simulink model "test_regler_polbvg_aktoren_sensoren_ansprechen"  (R2016b)
settings: Solver=ode1  StartTime=0.0  StopTime=Inf  FixedStep=0.001  RelTol=1e-3
PostLoadFcn:
  | , if any(exist('dsrtsu_mdlpostloadfcn', 'file') == [2, 3, 6]), try dsrtsu_mdlpostloadfcn('Execute', bdroot); catch fprintf('Error in PostLoadFcn (dsrtsu_mdlpostloadfcn) for model "%s":\n %s\n', bdroot, lasterr); end, end,
undefined symbols (not defined in the file): A_b_angle, A_D, B_b_angle, B_D, C_b_angle, C_D, Continuous, D_b_angle, D_D, matA_g, matA_hub_g, matB, matB_g, matB_hub, matB_hub_g, matC_g, matC_hub_g, matE, matE_hub, matR_ges, matR_hub, reglerhub, system, Time
libraries: rti1202lib_adc_class1 x3, rti1202lib_dac_class1 x2, ctrlSharedLib x2, simulink x1, rtiemclib x1, rti1202lib_base x1
(part 1 of 2)
PreSaveFcn:
  | , if any(exist('dsmpb_private', 'file') == [2, 3, 6]), try, dsmpb_private('dsmpb_mdlclblib', 'PreSave', bdroot); catch, disp(lasterr); end, end,
CloseFcn:
  | , if any(exist('dsmpb_private', 'file') == [2, 3, 6]), try, dsmpb_private('dsmpb_mdlclblib', 'Close', bdroot); catch, disp(lasterr); end, end,
settings Model: DSRTSU_INTERNAL_RTI_VER=490  DSRTSU_INTERNAL_RTI_TYPE=rti1202  DSRTSU_INTERNAL_RTIFPGA=80  DSMPB_DATASERVER_ModelPortLibVersion1=8  DSMPB_DATASERVER_DataServerVersion1=6  DSMPB_DATASERVER_DataServerStreamVersion1=3  ParamWorkspaceSource=ReferencedWorkspace  Creator=verladebruecke  LastModifiedBy=nicol
settings OptimizationCC: BlockReduction=off  OptimizeBlockIOStorage=off  BufferReuse=off  GlobalBufferReuse=off  ExpressionFolding=off  LocalBlockOutputs=off
settings HardwareCC: ProdBitPerPointer=32  ProdBitPerSizeT=32  ProdBitPerPtrDiffT=32  ProdLargestAtomicInteger=Integer  ProdEndianess=BigEndian  ProdWordSize=32  ProdHWDeviceType=Custom Processor->Custom  TargetIntDivRoundTo=Zero  TargetEndianess=BigEndian  TargetHWDeviceType=Custom Processor->Custom
settings RTWCC: SystemTargetFile=rti1202.tlc  MakeCommand=make_rti  TemplateMakefile=rti1202.tmf  Description=dSPACE DS1202 Hardware Platform
settings STFCustomTargetCC: ParMdlRefBuildCompliant=on  GRTInterface=off  SystemTargetFile=rti1202.tlc
settings GRTTargetCC: TargetLangStandard=C89/C90 (ANSI)  CompOptLevelCompliant=off  ConcurrentExecutionCompliant=off  CombineOutputUpdateFcns=off  MatFileLogging=off  CPPClassGenCompliant=off  UseToolchainInfoCompliant=off
settings ConfigComp: CovMetricSettings=dswe

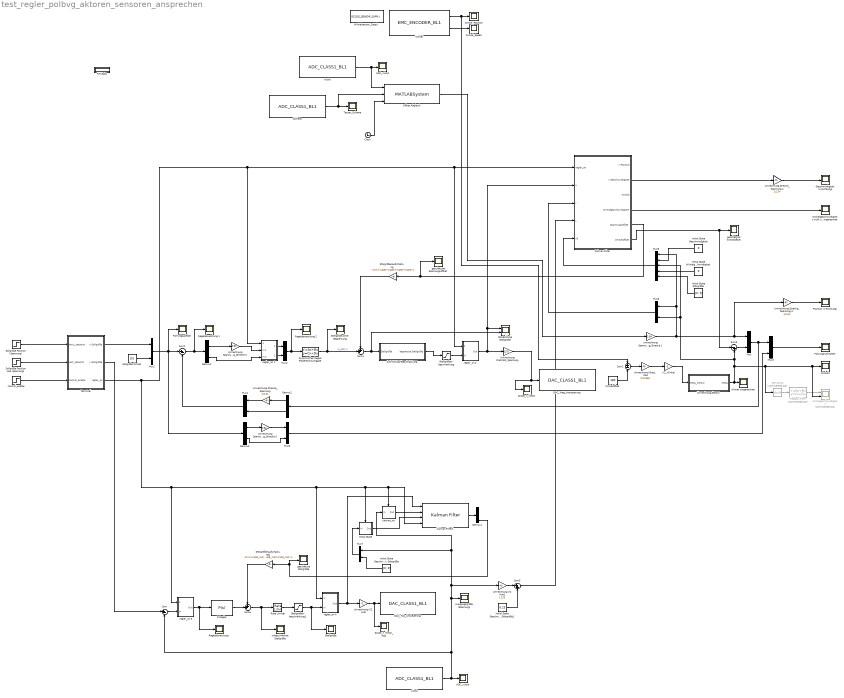
== system test_regler_polbvg_aktoren_sensoren_ansprechen ==
  ADC_xUout : Scope
  ADC_yUout : Scope
  Anti-Schlupf Beschränkung : Subsystem
  Ausgangsgröße (Spannung) : Scope
  Clock : Clock
  DAC_Hub_Ansteuerung : rti1202lib_dac_class1/DAC_CLASS1_BL1  DSProperties=struct('RTI',struct('Version',uint32(2),'BlockType',struct('isSLSource',uint8(0),'isSLSink',uint8(1),'isHWSource',uint8(0),'isHWSink',uint8(1),'isSetup',uint8(0),'isInline',uint8(1),'isNonInline',uint8(0),'isInterrupt',uint8(0),'isChannelwise',uint8(1)),'IOBoardType',{{'DS120X','STD','DACC1'}},'UnitType','DAC','Identifier','DAC','DialogType','ML','BlockSet','NONE','SlaveProcessor','NONE'))  RTIBlockInterface=struct('InputPortsActive',1,'InputPortsWidth',int32(1),'InputPortsDataType',{{'SS_DOUBLE'}},'InputPortsName',{{['DAC 2']}},'DialogFcn','rti120xstddacc1dacgui','InitLevel',3,'IconTransparency','on','BlockDisplay',{{['DAC CL1\nChannel: 2'],'center'}},'BlockName',struct('Token',{{'DAC_CLASS1_BL1'}}))  RTIBlockParameters=struct('ChannelNo',{{2,'OFF',[]}},'ChannelNumOf',{{1,'OFF',[]}},'InitialValue1',{{'0','OFF',[-10 10]}},'InitialValue2',{{'0','OFF',[-10 10]}},'InitialValue3',{{'0','OFF',[-10 10]}},'InitialValue4',{{'0','OFF',[-10 10]}},'InitialValue5',{{'0','OFF',[-10 10]}},'InitialValue6',{{'0','OFF',[-10 10]}},'InitialValue7',{{'0','OFF',[-10 10]}},'InitialValue8',{{'0','OFF',[-10 10]}},'InitialValue9',{{'0','OFF',[-10 10]}},'InitialValue10',{{'0','OFF',[-10 10]}},'InitialValue11',{{'0','OFF',[-10 10]}},'InitialValue12',{{'0','OFF',[-10 10]}},'InitialValue13',{{'0','OFF',[-10 10]}},'InitialValue14',{{'0','OFF',[-10 10]}},'InitialValue15',{{'0','OFF',[-10 10]}},'InitialValue16',{{'0','OFF',[-10 10]}},'OutputMode',{{[1 1 1 1 1 1 1 1 1 1 1 1 1 1 1 1],'OFF',[1 2]}},'TermValue1',{{'0','OFF',[-10 10]}},'TermValue2',{{'0','OFF',[-10 10]}},'TermValue3',{{'0','OFF',[-10 10]}},'TermValue4',{{'0','OFF',[-10 10]}},'TermValue5',{{'0','OFF',[-10 10]}},'TermValue6',{{'0','OFF',[-10 10]}},'TermValue7',{{'0','OFF',[-10 10]}},'TermValue8',{{'0','OFF',[-10 10]}},'TermValue9',{{'0','OFF',[-10 10]}},'TermValue10',{{'0','OFF',[-10 10]}},'TermValue11',{{'0','OFF',[-10 10]}},'TermValue12',{{'0','OFF',[-10 10]}},'TermValue13',{{'0','OFF',[-10 10]}},'TermValue14',{{'0','OFF',[-10 10]}},'TermValue15',{{'0','OFF',[-10 10]}},'TermValue16',{{'0','OFF',[-10 10]}},'EnableTermMode',{{0,'OFF',[0 1]}},'TLCFileName',{{'rti120xdac_c1_dac','OFF',[]}},'InitialValueBuildCheck1',{{0,'OFF',[]}},'InitialValueBuildCheck2',{{1,'OFF',[]}},'InitialValueBuildCheck3',{{0,'OFF',[]}},'InitialValueBuildCheck4',{{0,'OFF',[]}},'InitialValueBuildCheck5',{{0,'OFF',[]}},'InitialValueBuildCheck6',{{0,'OFF',[]}},'InitialValueBuildCheck7',{{0,'OFF',[]}},'InitialValueBuildCheck8',{{0,'OFF',[]}},'InitialValueBuildCheck9',{{0,'OFF',[]}},'InitialValueBuildCheck10',{{0,'OFF',[]}},'InitialValueBuildCheck11',{{0,'OFF',[]}},'InitialValueBuildCheck12',{{0,'OFF',[]}},'InitialValueBuildCheck13',{{0,'OFF',[]}},'InitialValueBuildCheck14',{{0,'OFF',[]}},'InitialValueBuildCheck15',{{0,'OFF',[]}},'InitialValueBuildCheck16',{{0,'OFF',[]}},'TermValueBuildCheck1',{{0,'OFF',[]}},'TermValueBuildCheck2',{{0,'OFF',[]}},'TermValueBuildCheck3',{{0,'OFF',[]}},'TermValueBuildCheck4',{{0,'OFF',[]}},'TermValueBuildCheck5',{{0,'OFF',[]}},'TermValueBuildCheck6',{{0,'OFF',[]}},'TermValueBuildCheck7',{{0,'OFF',[]}},'TermValueBuildCheck8',{{0,'OFF',[]}},'TermValueBuildCheck9',{{0,'OFF',[]}},'TermValueBuildCheck10',{{0,'OFF',[]}},'TermValueBuildCheck11',{{0,'OFF',[]}},'TermValueBuildCheck12',{{0,'OFF',[]}},'TermValueBuildCheck13',{{0,'OFF',[]}},'TermValueBuildCheck14',{{0,'OFF',[]}},'TermValueBuildCheck15',{{0,'OFF',[]}},'TermValueBuildCheck16',{{0,'OFF',[]}})  RTISFcnParameters=struct('ChannelNo','int16','ChannelNumOf','int16','InitialValue1','double','InitialValue2','double','InitialValue3','double','InitialValue4','double','InitialValue5','double','InitialValue6','double','InitialValue7','double','InitialValue8','double','InitialValue9','double','InitialValue10','double','InitialValue11','double','InitialValue12','double','InitialValue13','double','InitialValue14','double','InitialValue15','double','InitialValue16','double','OutputMode','int16','TermValue1','double','TermValue2','double','TermValue3','double','TermValue4','double','TermValue5','double','TermValue6','double','TermValue7','double','TermValue8','double','TermValue9','double','TermValue10','double','TermValue11','double','TermValue12','double','TermValue13','double','TermValue14','double','TermValue15','double','TermValue16','double','EnableTermMode','int16','TLCFileName','char')  RTIBlockParaDefault=struct('ChannelNo',1,'ChannelNumOf',1,'InitialValue1',0,'InitialValue2',0,'InitialValue3',0,'InitialValue4',0,'InitialValue5',0,'InitialValue6',0,'InitialValue7',0,'InitialValue8',0,'InitialValue9',0,'InitialValue10',0,'InitialValue11',0,'InitialValue12',0,'InitialValue13',0,'InitialValue14',0,'InitialValue15',0,'InitialValue16',0,'OutputMode',[1 1 1 1 1 1 1 1 1 1 1 1 1 1 1 1],'TermValue1',0,'TermValue2',0,'TermValue3',0,'TermValue4',0,'TermValue5',0,'TermValue6',0,'TermValue7',0,'TermValue8',0,'TermValue9',0,'TermValue10',0,'TermValue11',0,'TermValue12',0,'TermValue13',0,'TermValue14',0,'TermValue15',0,'TermValue16',0,'EnableTermMode',0,'TLCFileName','rti120xdac_c1_dac','InitialValueBuildCheck1',0,'InitialValueBuildCheck2',0,'InitialValueBuildCheck3',0,'InitialValueBuildCheck4',0,'InitialValueBuildCheck5',0,'InitialValueBuildCheck6',0,'InitialValueBuildCheck7',0,'InitialValueBuildCheck8',0,'InitialValueBuildCheck9',0,'InitialValueBuildCheck10',0,'InitialValueBuildCheck11',0,'InitialValueBuildCheck12',0,'InitialValueBuildCheck13',0,'InitialValueBuildCheck14',0,'InitialValueBuildCheck15',0,'InitialValueBuildCheck16',0,'TermValueBuildCheck1',0,'TermValueBuildCheck2',0,'TermValueBuildCheck3',0,'TermValueBuildCheck4',0,'TermValueBuildCheck5',0,'TermValueBuildCheck6',0,'TermValueBuildCheck7',0,'TermValueBuildCheck8',0,'TermValueBuildCheck9',0,'TermValueBuildCheck10',0,'TermValueBuildCheck11',0,'TermValueBuildCheck12',0,'TermValueBuildCheck13',0,'TermValueBuildCheck14',0,'TermValueBuildCheck15',0,'TermValueBuildCheck16',0)
  DAC_Weg_Ansteuerung : rti1202lib_dac_class1/DAC_CLASS1_BL1  DSProperties=struct('RTI',struct('Version',uint32(2),'BlockType',struct('isSLSource',uint8(0),'isSLSink',uint8(1),'isHWSource',uint8(0),'isHWSink',uint8(1),'isSetup',uint8(0),'isInline',uint8(1),'isNonInline',uint8(0),'isInterrupt',uint8(0),'isChannelwise',uint8(1)),'IOBoardType',{{'DS120X','STD','DACC1'}},'UnitType','DAC','Identifier','DAC','DialogType','ML','BlockSet','NONE','SlaveProcessor','NONE'))  RTIBlockInterface=struct('InputPortsActive',1,'InputPortsWidth',int32(1),'InputPortsDataType',{{'SS_DOUBLE'}},'InputPortsName',{{['DAC 1']}},'DialogFcn','rti120xstddacc1dacgui','InitLevel',3,'IconTransparency','on','BlockDisplay',{{['DAC CL1\nChannel: 1'],'center'}},'BlockName',struct('Token',{{'DAC_CLASS1_BL1'}}))  RTIBlockParameters=struct('ChannelNo',{{1,'OFF',[]}},'ChannelNumOf',{{1,'OFF',[]}},'InitialValue1',{{0,'OFF',[-10 10]}},'InitialValue2',{{0,'OFF',[-10 10]}},'InitialValue3',{{0,'OFF',[-10 10]}},'InitialValue4',{{0,'OFF',[-10 10]}},'InitialValue5',{{0,'OFF',[-10 10]}},'InitialValue6',{{0,'OFF',[-10 10]}},'InitialValue7',{{0,'OFF',[-10 10]}},'InitialValue8',{{0,'OFF',[-10 10]}},'InitialValue9',{{0,'OFF',[-10 10]}},'InitialValue10',{{0,'OFF',[-10 10]}},'InitialValue11',{{0,'OFF',[-10 10]}},'InitialValue12',{{0,'OFF',[-10 10]}},'InitialValue13',{{0,'OFF',[-10 10]}},'InitialValue14',{{0,'OFF',[-10 10]}},'InitialValue15',{{0,'OFF',[-10 10]}},'InitialValue16',{{0,'OFF',[-10 10]}},'OutputMode',{{[1 1 1 1 1 1 1 1 1 1 1 1 1 1 1 1],'OFF',[1 2]}},'TermValue1',{{0,'OFF',[-10 10]}},'TermValue2',{{0,'OFF',[-10 10]}},'TermValue3',{{0,'OFF',[-10 10]}},'TermValue4',{{0,'OFF',[-10 10]}},'TermValue5',{{0,'OFF',[-10 10]}},'TermValue6',{{0,'OFF',[-10 10]}},'TermValue7',{{0,'OFF',[-10 10]}},'TermValue8',{{0,'OFF',[-10 10]}},'TermValue9',{{0,'OFF',[-10 10]}},'TermValue10',{{0,'OFF',[-10 10]}},'TermValue11',{{0,'OFF',[-10 10]}},'TermValue12',{{0,'OFF',[-10 10]}},'TermValue13',{{0,'OFF',[-10 10]}},'TermValue14',{{0,'OFF',[-10 10]}},'TermValue15',{{0,'OFF',[-10 10]}},'TermValue16',{{0,'OFF',[-10 10]}},'EnableTermMode',{{0,'OFF',[0 1]}},'TLCFileName',{{'rti120xdac_c1_dac','OFF',[]}},'InitialValueBuildCheck1',{{0,'OFF',[]}},'InitialValueBuildCheck2',{{0,'OFF',[]}},'InitialValueBuildCheck3',{{0,'OFF',[]}},'InitialValueBuildCheck4',{{0,'OFF',[]}},'InitialValueBuildCheck5',{{0,'OFF',[]}},'InitialValueBuildCheck6',{{0,'OFF',[]}},'InitialValueBuildCheck7',{{0,'OFF',[]}},'InitialValueBuildCheck8',{{0,'OFF',[]}},'InitialValueBuildCheck9',{{0,'OFF',[]}},'InitialValueBuildCheck10',{{0,'OFF',[]}},'InitialValueBuildCheck11',{{0,'OFF',[]}},'InitialValueBuildCheck12',{{0,'OFF',[]}},'InitialValueBuildCheck13',{{0,'OFF',[]}},'InitialValueBuildCheck14',{{0,'OFF',[]}},'InitialValueBuildCheck15',{{0,'OFF',[]}},'InitialValueBuildCheck16',{{0,'OFF',[]}},'TermValueBuildCheck1',{{0,'OFF',[]}},'TermValueBuildCheck2',{{0,'OFF',[]}},'TermValueBuildCheck3',{{0,'OFF',[]}},'TermValueBuildCheck4',{{0,'OFF',[]}},'TermValueBuildCheck5',{{0,'OFF',[]}},'TermValueBuildCheck6',{{0,'OFF',[]}},'TermValueBuildCheck7',{{0,'OFF',[]}},'TermValueBuildCheck8',{{0,'OFF',[]}},'TermValueBuildCheck9',{{0,'OFF',[]}},'TermValueBuildCheck10',{{0,'OFF',[]}},'TermValueBuildCheck11',{{0,'OFF',[]}},'TermValueBuildCheck12',{{0,'OFF',[]}},'TermValueBuildCheck13',{{0,'OFF',[]}},'TermValueBuildCheck14',{{0,'OFF',[]}},'TermValueBuildCheck15',{{0,'OFF',[]}},'TermValueBuildCheck16',{{0,'OFF',[]}})  RTISFcnParameters=struct('ChannelNo','int16','ChannelNumOf','int16','InitialValue1','double','InitialValue2','double','InitialValue3','double','InitialValue4','double','InitialValue5','double','InitialValue6','double','InitialValue7','double','InitialValue8','double','InitialValue9','double','InitialValue10','double','InitialValue11','double','InitialValue12','double','InitialValue13','double','InitialValue14','double','InitialValue15','double','InitialValue16','double','OutputMode','int16','TermValue1','double','TermValue2','double','TermValue3','double','TermValue4','double','TermValue5','double','TermValue6','double','TermValue7','double','TermValue8','double','TermValue9','double','TermValue10','double','TermValue11','double','TermValue12','double','TermValue13','double','TermValue14','double','TermValue15','double','TermValue16','double','EnableTermMode','int16','TLCFileName','char')  RTIBlockParaDefault=struct('ChannelNo',1,'ChannelNumOf',1,'InitialValue1',0,'InitialValue2',0,'InitialValue3',0,'InitialValue4',0,'InitialValue5',0,'InitialValue6',0,'InitialValue7',0,'InitialValue8',0,'InitialValue9',0,'InitialValue10',0,'InitialValue11',0,'InitialValue12',0,'InitialValue13',0,'InitialValue14',0,'InitialValue15',0,'InitialValue16',0,'OutputMode',[1 1 1 1 1 1 1 1 1 1 1 1 1 1 1 1],'TermValue1',0,'TermValue2',0,'TermValue3',0,'TermValue4',0,'TermValue5',0,'TermValue6',0,'TermValue7',0,'TermValue8',0,'TermValue9',0,'TermValue10',0,'TermValue11',0,'TermValue12',0,'TermValue13',0,'TermValue14',0,'TermValue15',0,'TermValue16',0,'EnableTermMode',0,'TLCFileName','rti120xdac_c1_dac','InitialValueBuildCheck1',0,'InitialValueBuildCheck2',0,'InitialValueBuildCheck3',0,'InitialValueBuildCheck4',0,'InitialValueBuildCheck5',0,'InitialValueBuildCheck6',0,'InitialValueBuildCheck7',0,'InitialValueBuildCheck8',0,'InitialValueBuildCheck9',0,'InitialValueBuildCheck10',0,'InitialValueBuildCheck11',0,'InitialValueBuildCheck12',0,'InitialValueBuildCheck13',0,'InitialValueBuildCheck14',0,'InitialValueBuildCheck15',0,'InitialValueBuildCheck16',0,'TermValueBuildCheck1',0,'TermValueBuildCheck2',0,'TermValueBuildCheck3',0,'TermValueBuildCheck4',0,'TermValueBuildCheck5',0,'TermValueBuildCheck6',0,'TermValueBuildCheck7',0,'TermValueBuildCheck8',0,'TermValueBuildCheck9',0,'TermValueBuildCheck10',0,'TermValueBuildCheck11',0,'TermValueBuildCheck12',0,'TermValueBuildCheck13',0,'TermValueBuildCheck14',0,'TermValueBuildCheck15',0,'TermValueBuildCheck16',0)
  Demux1 : Demux  Outputs=2
  Demux2 : Demux  Outputs=2
  Demux3 : Demux  Outputs=2
  Demux4 : Demux  Outputs=3
  Derivative : Derivative  Commented=on
  Dynamischer Regler Polbereichsvorgabe : StateSpace  A=A_D  B=-B_D  C=-C_D  D=D_D  X0=0
  Führungsgrößen : Scope
  Führungsverhalten : Scope
  Geschwindigkeit (x-Richtung) : Scope
  Initial State : Subsystem  TreatAsAtomicUnit=on
  Initial State Geschwindigkeit : Constant  Value=0  VectorParams1D=off
  "Initial State Geschwindigkeit, Störgröße" : Constant  Value=[0; 0]  VectorParams1D=off
  "Initial State Geschwindigkeit, Störgröße1" : Constant  Value=0.23  VectorParams1D=off
  Initial State Störgröße : Constant  Value=[0; 0]  VectorParams1D=off
  Initial State Winkelgeschwindigkeit : Constant  Value=0  VectorParams1D=off
  Kalman Filter : Subsystem
  Kalman Filter1 : ctrlSharedLib/Kalman Filter  TimeDomain=Continuous-Time  UseCurrentEstimator=on  ModelSource=Individual A, B, C, D matrices  ModelSourceVariable=ss(0.95,1,1,0,1)  A=matA_hub_g  B=matB_hub_g  C=matC_hub_g  D=0  NumberOfStates=1  NumberOfInputs=1  NumberOfOutputs=1  InitialEstimateSource=Input port  X0=0  P0=10  UseK=off  UseGH=on  NumberOfProcessNoiseInputs=1  G=matG_hub  TimeInvariantG=on  H=0  TimeInvariantH=on  Q=matQ_hub  TimeInvariantQ=on  R=matR_hub  TimeInvariantR=on  N=0  TimeInvariantN=on  AddInputPort=on  AddEnablePort=off  ExternalReset=rising  OutputEstimatedY=off  OutputP=off  Ts=-1
  Mux{,1..5,7..8} (8 alike) : Mux  Inputs=2
  Mux6 : Mux  Inputs=5
  Offset Abgleich : MATLABSystem  System=offset_abgleich  SimulateUsing=Code generation
      mask Type: offset_abgleich
      mask Display:
      | disp('offset_abgleich');
      | port_label('input',1,'input');
      | port_label('input',2,'taster');
      | port_label('input',3,'clock');
      | port_label('output',1,'output');
  P-Regler : simulink/Continuous/PID Controller  Controller=P  TimeDomain=Continuous-time  SampleTime=-1  IntegratorMethod=Forward Euler  FilterMethod=Forward Euler  Form=Parallel  UseFilter=on  ControllerParametersSource=internal  P=reglerhub.P  I=0  D=0.1  N=100  InitialConditionSource=internal  InitialConditionForIntegrator=0  InitialConditionForFilter=0  ExternalReset=falling  LimitOutput=off  UpperSaturationLimit=inf  LowerSaturationLimit=-inf  LinearizeAsGain=on  AntiWindupMode=none  Kb=1  TrackingMode=on  Kt=2  PParamMin=[]  PParamMax=[]  IParamMin=[]  IParamMax=[]  DParamMin=[]  DParamMax=[]  NParamMin=[]  NParamMax=[]  KbParamMin=[]  KbParamMax=[]  KtParamMin=[]  KtParamMax=[]  POutMin=[]  POutMax=[]  IOutMin=[]  IOutMax=[]  DOutMin=[]  DOutMax=[]  NOutMin=[]  NOutMax=[]  KbOutMin=[]  KbOutMax=[]  KtOutMin=[]  KtOutMax=[]  IntegratorOutMin=[]  IntegratorOutMax=[]  FilterOutMin=[]  FilterOutMax=[]  SumOutMin=[]  SumOutMax=[]  SumI1OutMin=[]  SumI1OutMax=[]  SumI2OutMin=[]  SumI2OutMax=[]  SumI3OutMin=[]  SumI3OutMax=[]  SumDOutMin=[]  SumDOutMax=[]  SaturationOutMin=[]  SaturationOutMax=[]  IntegratorContinuousStateAttributes=''  IntegratorStateMustResolveToSignalObject=off  IntegratorRTWStateStorageClass=Auto  FilterContinuousStateAttributes=''  FilterStateMustResolveToSignalObject=off  FilterRTWStateStorageClass=Auto  DifferentiatorICPrevScaledInput=0  DifferentiatorOutMin=[]  DifferentiatorOutMax=[]
  Position (x-Richtung) : Scope
  RTI Data : Subsystem  Tag=struct('RTIDataServer',struct('RTIDataServerVs','2','RTIModelDescription','struct(''main'',''aktoren_sensoren_ansprechen'',''sub'','''',''isMp'',0)'))  LoadFcn="if exist('rtidc'), try,  rtidc('DataHostBlockClbLoad', gcbh); catch, disp(['Warning: ''LoadFcn'' for RTI Data block failed: ' lasterr]); end, end,"  mask(RTI_DATA_HOST){}
      mask help:
      | RTI Data Block.
      | This block is used by RTI to store internal model-dependent data.
      | Please keep this block on the root level of the model. Deleting this block will result in data loss.
      |
      | NEVER DELETE OR COPY THIS BLOCK!
      settings: CopyFcn="if exist('rtidc'), try,  rtidc('DataHostBlockClbCopy', gcbh); catch, disp(['Warning: ''CopyFcn'' for RTI Data block failed: ' lasterr]); end, end,"  DeleteFcn="if exist('rtidc'), try,  rtidc('DataHostBlockClbDelete', gcbh); catch, disp(['Warning: ''DeleteFcn'' for RTI Data block failed: ' lasterr]); end, end,"  ModelCloseFcn="if exist('rtidc'), try,  rtidc('DataHostBlockClbModelClose', gcbh); catch, disp(['Warning: ''ModelCloseFcn'' for RTI Data block failed: ' lasterr]); end, end,"  PreSaveFcn="if exist('rtidc'), try,  rtidc('DataHostBlockClbPreSave', gcbh); catch, disp(['Warning: ''PreSaveFcn'' for RTI Data block failed: ' lasterr]); end, end,"  PostSaveFcn="if exist('rtidc'), try,  rtidc('DataHostBlockClbPostSave', gcbh); catch, disp(['Warning: ''PostSaveFcn'' for RTI Data block failed: ' lasterr]); end, end,"  NameChangeFcn="if exist('rtidc'), try,  rtidc('DataHostBlockClbNameChange', gcbh); catch, disp(['Warning: ''NameChangeFcn'' for RTI Data block failed: ' lasterr]); end, end,"
      mask Help:
      | RTI Data Block.
      | This block is used by RTI to store internal model-dependent data.
      | Please keep this block on the root level of the model. Deleting this block will result in data loss.
      | 
      | NEVER DELETE OR COPY THIS BLOCK!
      mask Display:
      | text(0.5, 0.5, 'RTI Data', 'HorizontalAlignment', 'center');
      | plot([1 0]);
  Rate Limiter : RateLimiter  RisingSlewLimit=0.23024  FallingSlewLimit=-0.23024  SampleTimeMode=inherited
  Regelabweichung : Scope
  Regelabweichung 1 : Scope
  Regelabweichung 2 : Scope
  Schiene : rti1202lib_adc_class1/ADC_CLASS1_BL1  DSProperties=struct('RTI',struct('Version',uint32(1),'BlockType',struct('isSLSource',uint8(1),'isSLSink',uint8(1),'isHWSource',uint8(0),'isHWSink',uint8(1),'isSetup',uint8(0),'isInline',uint8(1),'isNonInline',uint8(0),'isInterrupt',uint8(0),'isChannelwise',uint8(1)),'IOBoardType',{{'DS120X','STD','ADCC1'}},'UnitType','ADC','Identifier','ADC','DialogType','ML','BlockSet','NONE','SlaveProcessor','NONE'))  RTIBlockInterface=struct('InputPortsActive',0,'InputPortsWidth',int32(1),'InputPortsDataType',{{'SS_BOOLEAN'}},'InputPortsName',{{'Continue'}},'OutputPortsActive',[1 0],'OutputPortsWidth',int32([1 1]),'OutputPortsDataType',{{'SS_DOUBLE','SS_INT16'}},'OutputPortsName',{{'ADC','Status'}},'DialogFcn','rti120xstdadcc1adcgui','SampleTime',{{-1}},'InitLevel',3,'IconTransparency','on','BlockDisplay',{{['ADC CL1\nChannel: 10'],'center'}},'BlockName',struct('Token',{{'ADC_CLASS1_BL1'}}))  RTIBlockParameters=struct('ReadMode',{{1,'OFF',[1 2]}},'ChannelNo',{{10,'OFF',[]}},'ConversionMode',{{1,'OFF',[1 2]}},'TriggerSource',{{1,'OFF',[1 2]}},'TriggerLineIn',{{1,'OFF',[1 16]}},'SampleMode',{{1,'OFF',[1 2]}},'BurstTriggerSource',{{1,'OFF',[1 2]}},'BurstTriggerLine',{{1,'OFF',[1 16]}},'ConvTriggerSource',{{3,'OFF',[1 3]}},'ConvTriggerLine',{{1,'OFF',[1 16]}},'ConvPeriod',{{'100e-6','OFF',[1e-06 1.34]}},'ConvPeriodCheck',{{0,'OFF',[]}},'BurstSize',{{'10','OFF',[]}},'BurstSizeCheck',{{0,'OFF',[]}},'DataSetOffset',{{'0','OFF',[]}},'DataSetOffsetCheck',{{0,'OFF',[]}},'DataSetLength',{{'1','OFF',[]}},'DataSetLengthCheck',{{0,'OFF',[]}},'EnableTriggerEvent',{{0,'OFF',[0 1]}},'TriggerMode',{{2,'OFF',[1 3]}},'TriggerLineOut',{{1,'OFF',[1 16]}},'ADCSWStartEnable',{{0,'OFF',[0 1]}},'SampleTime',{{'-1','OFF',[-1 inf]}},'SampleTimeCheck',{{1,'OFF',[]}},'StatusPortEnable',{{0,'OFF',[0 1]}},'TLCFileName',{{'rti120xadc_c1_adc','OFF',[]}})  RTISFcnParameters=struct('ReadMode','int16','ChannelNo','int16','ConversionMode','int16','TriggerSource','int16','TriggerLineIn','int16','SampleMode','int16','BurstTriggerSource','int16','BurstTriggerLine','int16','ConvTriggerSource','int16','ConvTriggerLine','int16','ConvPeriod','double','BurstSize','int16','DataSetOffset','int16','DataSetLength','int16','EnableTriggerEvent','int16','TriggerMode','int16','TriggerLineOut','int16','ADCSWStartEnable','int16','SampleTime','double','StatusPortEnable','int16','TLCFileName','char')  RTIBlockParaDefault=struct('ReadMode',1,'ChannelNo',1,'ConversionMode',1,'TriggerSource',1,'TriggerLineIn',1,'SampleMode',1,'BurstTriggerSource',1,'BurstTriggerLine',1,'ConvTriggerSource',3,'ConvTriggerLine',1,'ConvPeriod',0.0001,'ConvPeriodCheck',0,'BurstSize',10,'BurstSizeCheck',0,'DataSetOffset',0,'DataSetOffsetCheck',0,'DataSetLength',1,'DataSetLengthCheck',0,'EnableTriggerEvent',0,'TriggerMode',2,'TriggerLineOut',1,'ADCSWStartEnable',0,'SampleTime',-1,'SampleTimeCheck',1,'StatusPortEnable',0,'TLCFileName','rti120xadc_c1_adc')
  Scope_n_Motor : Scope
  Scope_n_Motor_Hub : Scope
  Sollgröße Position (Spannung) : Step  Time=2  SampleTime=0
  Sollgröße Position Hub (Spannung) : Step  Time=2  After=0.5  SampleTime=0
  Sollgröße Winkel : Constant  Value=[0]  VectorParams1D=off
  Stellgröße : Scope
  Stellgröße ohne Begrenzung : Scope
  Stellgrößen- beschränkung : Saturate  UpperLimit=75  LowerLimit=-75
  Stellgrößen- beschränkung1 : Saturate  UpperLimit=1  LowerLimit=-1
  Störgrößenaufschaltung : Gain  Gain=-1*inv(matB'*matB)*matB'*matE  Multiplication=Matrix(K*u)
  Störgrößenaufschaltung1 : Gain  Gain=-1*inv(matB_hub'*matB_hub)*matB_hub'*matE_hub  Multiplication=Matrix(K*u)
  Sum : Sum  Inputs=|+-
  Sum1 : Sum  Inputs=|+-
  Sum2 : Sum  Inputs=+|-
  Sum3 : Sum  Inputs=|-+
  Sum4 : Sum  Inputs=++|
  Sum5 : Sum  Inputs=|++
  Sum6 : Sum  Inputs=++|
  Taster_Schiene : Scope
  Terminal : Subsystem
  Tiefpass Filter : StateSpace  Commented=on  A=A_b_angle  B=B_b_angle  C=C_b_angle  D=D_b_angle  X0=0
  Umrechnung Drehzahl_Spannung : Gain  Gain=1/75
  Umrechnung Grad_Rad : Gain  Gain=2*pi/360
  Umrechnung Spannung_Strecke 1 : Gain  Gain=2.54
  Umrechnung Spannung_Strecke 2 : Gain  Gain=2.54
  Umrechnung Spannung_Strecke 3 : Gain  Gain=2.54
  Umrechnung Strecke_Spannung : Gain  Gain=1/2.54
  Umrechnung Strecke_Spannung 3 : Gain  Gain=1/2.54
  Umrechnung Strecke_Spannung 4 : Gain  Gain=1/2.54
  Umrechnung VZ Hub : Gain  Gain=-1
  Umrechnung VZ Hub1 : Gain  Gain=1.375
  Umrechnung Sensor : MATLAB Function  TreatAsAtomicUnit=on
  VZ_Winkel : Gain  Gain=-1
  Winkel : rtiemclib/EMC_ENCODER_BL1  DSProperties=struct('RTI',struct('Version',uint32(1),'BlockType',struct('isSLSource',uint8(1),'isSLSink',uint8(0),'isHWSource',uint8(1),'isHWSink',uint8(0),'isSetup',uint8(0),'isInline',uint8(1),'isNonInline',uint8(0),'isInterrupt',uint8(0),'isChannelwise',uint8(1)),'IOBoardType','DSEMC','UnitType','ENCODER','Identifier','ENCODER','DialogType','ML','BlockSet','RTIEMC','SlaveProcessor','NONE'))  RTIBlockInterface=struct('OutputPortsWidth',int32([1 1 1]),'OutputPortsActive',int32([1 1 0]),'OutputPortsName',{{'Position','Speed',['Index Detected']}},'OutputPortsDataType',{{'SS_DOUBLE','SS_DOUBLE','SS_BOOLEAN'}},'InitLevel',3,'IconTransparency','on','BlockDisplay',{{['EMC Encoder\nUnit: 1\nDIO class: 2\nPort: 1\nChannel: 1'],'center'}},'DialogFcn','rtiemcencodergui','BlockName',struct('Token',{{'EMC_ENCODER_BL1'}}))  RTIBlockParameters=struct('UnitNo',{{1,'OFF',[1 6]}},'DioClassNo',{{2,'OFF',[1 2]}},'PortNo',{{1,'OFF',[1 1]}},'ChannelNo',{{1,'OFF',[1 11]}},'HwSignalPin',{{['DIO1 ch1'],'OFF',[]}},'HwRefPin',{{'GND','OFF',[]}},'EnablePosMeasurement',{{0,'OFF',[0 1]}},'IndexSetMode',{{1,'OFF',[1 3]}},'NumOfLines',{{'1024','OFF',[1 2097152]}},'InitAngleValue',{{'180','OFF',[0 359.99999]}},'IndexAngleValue',{{'0','OFF',[0 359.99999]}},'MinPosValue',{{'0','OFF',[-2097152 2097150.75]}},'MaxPosValue',{{'1023.75','OFF',[-2097151 2097151.75]}},'InitPosValue',{{'0','OFF',[-2097152 2097151.75]}},'IndexPosValue',{{'0','OFF',[-2097152 2097151.75]}},'IndexGateMode',{{0,'OFF',[0 1]}},'EnableNoiseFilter',{{0,'OFF',[0 1]}},'FilterInterval',{{'0','OFF',[0 0.01]}},'IndexDetectedOutPortMode',{{0,'OFF',[0 1]}},'BuildCheckAngleMeasurement',{{1,'OFF',[0 1]}},'BuildCheckAngleIndexMode',{{0,'OFF',[0 1]}},'BuildCheckPosIndexMode',{{0,'OFF',[0 1]}},'TLCFileName',{{'rtiemcencoder','OFF',[]}})  RTISFcnParameters=struct('UnitNo','int32','DioClassNo','int32','PortNo','int32','ChannelNo','int32','EnablePosMeasurement','int32','IndexSetMode','int32','IndexDetectedOutPortMode','int32','NumOfLines','uint32','InitAngleValue','double','IndexAngleValue','double','MinPosValue','double','MaxPosValue','double','InitPosValue','double','IndexPosValue','double','IndexGateMode','int32','EnableNoiseFilter','int32','FilterInterval','double','TLCFileName','char')  RTIBlockParaDefault=struct('UnitNo',1,'DioClassNo',1,'PortNo',1,'ChannelNo',1,'HwSignalPin',['DIO1 ch1'],'HwRefPin','GND','EnablePosMeasurement',0,'IndexSetMode',1,'NumOfLines',1024,'InitAngleValue',60,'IndexAngleValue',0,'MinPosValue',0,'MaxPosValue',1023.75,'InitPosValue',0,'IndexPosValue',0,'IndexGateMode',0,'EnableNoiseFilter',0,'FilterInterval',0,'IndexDetectedOutPortMode',0,'BuildCheckAngleMeasurement',0,'BuildCheckAngleIndexMode',0,'BuildCheckPosIndexMode',0,'TLCFileName','rtiemcencoder')
  Winkel umgerechnet : Scope
  Winkel1 : Scope
  Winkel_Position : Scope
  Winkel_Speed : Scope
  Winkelgeschwindigkeit : Scope  Commented=on  NumInputPorts=2
  Winkelgeschwindigkeit nicht umgerechnet : Scope
  Winkeloffset : Constant  Value=180
  Winkelsensor_Supply : rti1202lib_base/DS1202_SENSOR_SUPPLY  DSProperties=struct('RTI',struct('Version',uint32(1),'BlockType',struct('isSLSource',uint8(0),'isSLSink',uint8(0),'isHWSource',uint8(0),'isHWSink',uint8(1),'isSetup',uint8(0),'isInline',uint8(1),'isNonInline',uint8(0),'isInterrupt',uint8(0),'isChannelwise',uint8(0)),'IOBoardType',{{'DS120X','BASE'}},'UnitType','SENSORSUPPLY','Identifier','SENSORSUPPLY','DialogType','ML','BlockSet','NONE','SlaveProcessor','NONE'))  RTIBlockInterface=struct('OutputPortsActive',0,'OutputPortsWidth',int32(0),'DialogFcn','rti120xbasesensorsupplygui','InitLevel',3,'IconTransparency','off','BlockDisplay',{{['DS1202\nSensor Supply'],'center'}},'BlockName',struct('Token',{{'DS1202_SENSOR_SUPPLY'}}))  RTIBlockParameters=struct('Voltage',{{'5','OFF',[2 20]}},'TLCFileName',{{'rti120xbase_sensor_supply','OFF',[]}})  RTISFcnParameters=struct('Voltage','int16','TLCFileName','char')  RTIBlockParaDefault=struct('Voltage',2,'TLCFileName','rti120xbase_sensor_supply')
  control_enable : Step  Time=2  SampleTime=0
  geschätzte Störgröße : Scope
  geschätzter Spannungsoffset : Scope
  geschätzter Winkeloffset : Scope
  kalman_on : Subsystem  TreatAsAtomicUnit=on
  regler_on 1 : Subsystem
  regler_on 2 : Subsystem
  regler_on 3 : Subsystem
  regler_on 4 : Subsystem
  tatsächliche Stellgröße : Scope  NumInputPorts=2
  unbeschränkte Stellgröße : Scope
  xUout : rti1202lib_adc_class1/ADC_CLASS1_BL1  DSProperties=struct('RTI',struct('Version',uint32(1),'BlockType',struct('isSLSource',uint8(1),'isSLSink',uint8(1),'isHWSource',uint8(0),'isHWSink',uint8(1),'isSetup',uint8(0),'isInline',uint8(1),'isNonInline',uint8(0),'isInterrupt',uint8(0),'isChannelwise',uint8(1)),'IOBoardType',{{'DS120X','STD','ADCC1'}},'UnitType','ADC','Identifier','ADC','DialogType','ML','BlockSet','NONE','SlaveProcessor','NONE'))  RTIBlockInterface=struct('InputPortsActive',0,'InputPortsWidth',int32(1),'InputPortsDataType',{{'SS_BOOLEAN'}},'InputPortsName',{{'Continue'}},'OutputPortsActive',[1 0],'OutputPortsWidth',int32([1 1]),'OutputPortsDataType',{{'SS_DOUBLE','SS_INT16'}},'OutputPortsName',{{'ADC','Status'}},'DialogFcn','rti120xstdadcc1adcgui','SampleTime',{{-1}},'InitLevel',3,'IconTransparency','on','BlockDisplay',{{['ADC CL1\nChannel: 1'],'center'}},'BlockName',struct('Token',{{'ADC_CLASS1_BL1'}}))  RTIBlockParameters=struct('ReadMode',{{1,'OFF',[1 2]}},'ChannelNo',{{1,'OFF',[]}},'ConversionMode',{{1,'OFF',[1 2]}},'TriggerSource',{{1,'OFF',[1 2]}},'TriggerLineIn',{{1,'OFF',[1 16]}},'SampleMode',{{1,'OFF',[1 2]}},'BurstTriggerSource',{{1,'OFF',[1 2]}},'BurstTriggerLine',{{1,'OFF',[1 16]}},'ConvTriggerSource',{{3,'OFF',[1 3]}},'ConvTriggerLine',{{1,'OFF',[1 16]}},'ConvPeriod',{{'100e-6','OFF',[1e-06 1.34]}},'ConvPeriodCheck',{{0,'OFF',[]}},'BurstSize',{{'10','OFF',[]}},'BurstSizeCheck',{{0,'OFF',[]}},'DataSetOffset',{{'0','OFF',[]}},'DataSetOffsetCheck',{{0,'OFF',[]}},'DataSetLength',{{'1','OFF',[]}},'DataSetLengthCheck',{{0,'OFF',[]}},'EnableTriggerEvent',{{0,'OFF',[0 1]}},'TriggerMode',{{2,'OFF',[1 3]}},'TriggerLineOut',{{1,'OFF',[1 16]}},'ADCSWStartEnable',{{0,'OFF',[0 1]}},'SampleTime',{{'-1','OFF',[-1 inf]}},'SampleTimeCheck',{{1,'OFF',[]}},'StatusPortEnable',{{0,'OFF',[0 1]}},'TLCFileName',{{'rti120xadc_c1_adc','OFF',[]}})  RTISFcnParameters=struct('ReadMode','int16','ChannelNo','int16','ConversionMode','int16','TriggerSource','int16','TriggerLineIn','int16','SampleMode','int16','BurstTriggerSource','int16','BurstTriggerLine','int16','ConvTriggerSource','int16','ConvTriggerLine','int16','ConvPeriod','double','BurstSize','int16','DataSetOffset','int16','DataSetLength','int16','EnableTriggerEvent','int16','TriggerMode','int16','TriggerLineOut','int16','ADCSWStartEnable','int16','SampleTime','double','StatusPortEnable','int16','TLCFileName','char')  RTIBlockParaDefault=struct('ReadMode',1,'ChannelNo',1,'ConversionMode',1,'TriggerSource',1,'TriggerLineIn',1,'SampleMode',1,'BurstTriggerSource',1,'BurstTriggerLine',1,'ConvTriggerSource',3,'ConvTriggerLine',1,'ConvPeriod',0.0001,'ConvPeriodCheck',0,'BurstSize',10,'BurstSizeCheck',0,'DataSetOffset',0,'DataSetOffsetCheck',0,'DataSetLength',1,'DataSetLengthCheck',0,'EnableTriggerEvent',0,'TriggerMode',2,'TriggerLineOut',1,'ADCSWStartEnable',0,'SampleTime',-1,'SampleTimeCheck',1,'StatusPortEnable',0,'TLCFileName','rti120xadc_c1_adc')
  yUout : rti1202lib_adc_class1/ADC_CLASS1_BL1  DSProperties=struct('RTI',struct('Version',uint32(1),'BlockType',struct('isSLSource',uint8(1),'isSLSink',uint8(1),'isHWSource',uint8(0),'isHWSink',uint8(1),'isSetup',uint8(0),'isInline',uint8(1),'isNonInline',uint8(0),'isInterrupt',uint8(0),'isChannelwise',uint8(1)),'IOBoardType',{{'DS120X','STD','ADCC1'}},'UnitType','ADC','Identifier','ADC','DialogType','ML','BlockSet','NONE','SlaveProcessor','NONE'))  RTIBlockInterface=struct('InputPortsActive',0,'InputPortsWidth',int32(1),'InputPortsDataType',{{'SS_BOOLEAN'}},'InputPortsName',{{'Continue'}},'OutputPortsActive',[1 0],'OutputPortsWidth',int32([1 1]),'OutputPortsDataType',{{'SS_DOUBLE','SS_INT16'}},'OutputPortsName',{{'ADC','Status'}},'DialogFcn','rti120xstdadcc1adcgui','SampleTime',{{-1}},'InitLevel',3,'IconTransparency','on','BlockDisplay',{{['ADC CL1\nChannel: 2'],'center'}},'BlockName',struct('Token',{{'ADC_CLASS1_BL1'}}))  RTIBlockParameters=struct('ReadMode',{{1,'OFF',[1 2]}},'ChannelNo',{{2,'OFF',[]}},'ConversionMode',{{1,'OFF',[1 2]}},'TriggerSource',{{1,'OFF',[1 2]}},'TriggerLineIn',{{1,'OFF',[1 16]}},'SampleMode',{{1,'OFF',[1 2]}},'BurstTriggerSource',{{1,'OFF',[1 2]}},'BurstTriggerLine',{{1,'OFF',[1 16]}},'ConvTriggerSource',{{3,'OFF',[1 3]}},'ConvTriggerLine',{{1,'OFF',[1 16]}},'ConvPeriod',{{'100e-6','OFF',[1e-06 1.34]}},'ConvPeriodCheck',{{0,'OFF',[]}},'BurstSize',{{'10','OFF',[]}},'BurstSizeCheck',{{0,'OFF',[]}},'DataSetOffset',{{'0','OFF',[]}},'DataSetOffsetCheck',{{0,'OFF',[]}},'DataSetLength',{{'1','OFF',[]}},'DataSetLengthCheck',{{0,'OFF',[]}},'EnableTriggerEvent',{{0,'OFF',[0 1]}},'TriggerMode',{{2,'OFF',[1 3]}},'TriggerLineOut',{{1,'OFF',[1 16]}},'ADCSWStartEnable',{{0,'OFF',[0 1]}},'SampleTime',{{'-1','OFF',[-1 inf]}},'SampleTimeCheck',{{1,'OFF',[]}},'StatusPortEnable',{{0,'OFF',[0 1]}},'TLCFileName',{{'rti120xadc_c1_adc','OFF',[]}})  RTISFcnParameters=struct('ReadMode','int16','ChannelNo','int16','ConversionMode','int16','TriggerSource','int16','TriggerLineIn','int16','SampleMode','int16','BurstTriggerSource','int16','BurstTriggerLine','int16','ConvTriggerSource','int16','ConvTriggerLine','int16','ConvPeriod','double','BurstSize','int16','DataSetOffset','int16','DataSetLength','int16','EnableTriggerEvent','int16','TriggerMode','int16','TriggerLineOut','int16','ADCSWStartEnable','int16','SampleTime','double','StatusPortEnable','int16','TLCFileName','char')  RTIBlockParaDefault=struct('ReadMode',1,'ChannelNo',1,'ConversionMode',1,'TriggerSource',1,'TriggerLineIn',1,'SampleMode',1,'BurstTriggerSource',1,'BurstTriggerLine',1,'ConvTriggerSource',3,'ConvTriggerLine',1,'ConvPeriod',0.0001,'ConvPeriodCheck',0,'BurstSize',10,'BurstSizeCheck',0,'DataSetOffset',0,'DataSetOffsetCheck',0,'DataSetLength',1,'DataSetLengthCheck',0,'EnableTriggerEvent',0,'TriggerMode',2,'TriggerLineOut',1,'ADCSWStartEnable',0,'SampleTime',-1,'SampleTimeCheck',1,'StatusPortEnable',0,'TLCFileName','rti120xadc_c1_adc')
  wires:
  Winkel/2 -> Winkel_Speed/1
  Umrechnung Drehzahl_Spannung/1 -> Scope_n_Motor/1, DAC_Weg_Ansteuerung/1
  Dynamischer Regler Polbereichsvorgabe/1 -> Sum4/2, Stellgröße ohne Begrenzung/1  "U_soll; u"
  Mux/1 -> Demux2/1, Mux3/1
  Sollgröße Winkel/1 -> Mux2/2
  Mux3/1 -> Führungsverhalten/1
  Sum2/1 -> Umrechnung Grad_Rad/1
  Winkeloffset/1 -> Sum2/2
  Umrechnung Grad_Rad/1 -> VZ_Winkel/1
  VZ_Winkel/1 -> Umrechnung Sensor/1(theta_sensor)
  Anti-Schlupf Beschränkung/1(begrenzte Stellgröße) -> Stellgrößen- beschränkung/1
  Demux2/1 -> Umrechnung Strecke_Spannung/1
  Umrechnung Strecke_Spannung/1 -> Mux1/1
  Demux2/2 -> Mux1/2
  Umrechnung Spannung_Strecke 2/1 -> regler_on 1/2(In 1)
  Demux1/1 -> Umrechnung Spannung_Strecke 2/1
  Demux1/2 -> regler_on 1/3(In 2)
  Sum1/1 -> Demux1/1, Regelabweichung 1/1
  Umrechnung Spannung_Strecke 3/1 -> Mux5/1
  Demux3/1 -> Umrechnung Spannung_Strecke 3/1
  Demux3/2 -> Mux5/2
  Mux2/1 -> Sum1/1, Führungsgrößen/1, Demux3/1
  Mux5/1 -> Mux3/2
  Mux1/1 -> Sum1/2
  Winkel/1 -> Sum2/1, Winkel_Position/1
  Sum4/1 -> tatsächliche Stellgröße/2, Anti-Schlupf Beschränkung/1(Stellgröße)
  Offset Abgleich/1 -> Umrechnung Spannung_Strecke 1/1
  Umrechnung Spannung_Strecke 1/1 -> Mux8/1, Mux6/1, Umrechnung Strecke_Spannung 3/1, Mux/1
  regler_on 1/2(Out 2) -> Mux4/2
  regler_on 1/1(Out 1) -> Mux4/1
  Mux4/1 -> Regelabweichung 2/1, Dynamischer Regler Polbereichsvorgabe/1
  Stellgrößen- beschränkung/1 -> regler_on 2/2(In)
  Derivative/1 -> Tiefpass Filter/1
  Tiefpass Filter/1 -> Winkelgeschwindigkeit/1
  Sollgröße Position (Spannung)/1 -> Terminal/1(horiz_setpoint)
  control_enable/1 -> Terminal/3(control_enable)
  Sollgröße Position Hub (Spannung)/1 -> Terminal/2(vert_setpoint)
  Terminal/1(x-Sollgröße) -> Mux2/1
  Störgrößenaufschaltung/1 -> Sum4/1
  Umrechnung Strecke_Spannung 3/1 -> Position (x-Richtung)/1
  Kalman Filter/2(x-Geschwindigkeit) -> Umrechnung Strecke_Spannung 4/1
  Sum3/1 -> Mux/2
  regler_on 2/1(Out) -> Umrechnung Drehzahl_Spannung/1, Kalman Filter/2(u), tatsächliche Stellgröße/1
  Kalman Filter/5(Spannungsoffset) -> geschätzter Spannungsoffset/1, Störgrößenaufschaltung/1
  Mux6/1 -> Kalman Filter/5(x0)
  Mux8/1 -> Kalman Filter/3(y)
  Kalman Filter/6(Winkeloffset) -> Sum3/1, geschätzter Winkeloffset/1
  Kalman Filter/4(Winkelgeschwindigkeit) -> Winkelgeschwindigkeit nicht umgerechnet/1
  Initial State Störgröße/1 -> Mux6/5
  Initial State Winkelgeschwindigkeit/1 -> Mux6/4
  Initial State Geschwindigkeit/1 -> Mux6/2
  Umrechnung Strecke_Spannung 4/1 -> Geschwindigkeit (x-Richtung)/1
  Umrechnung Sensor/1(theta) -> Derivative/1, Winkelgeschwindigkeit/2, Winkel1/1, Mux8/2, Mux6/3, Sum3/2, Winkel umgerechnet/1
  xUout/1 -> Offset Abgleich/1, ADC_xUout/1
  Clock/1 -> Offset Abgleich/3
  Schiene/1 -> Offset Abgleich/2, Taster_Schiene/1
  Rate Limiter/1 -> Stellgrößen- beschränkung1/1
  Stellgrößen- beschränkung1/1 -> regler_on 4/2(In), Stellgröße/1
  Terminal/2(y-Sollgröße) -> Sum/1
  regler_on 4/1(Out) -> Kalman Filter1/1, Umrechnung VZ Hub/1
  regler_on 3/1(Out) -> Regelabweichung/1, P-Regler/1
  Sum/1 -> regler_on 3/2(In)
  P-Regler/1 -> Sum6/2
  Sum6/1 -> Rate Limiter/1, unbeschränkte Stellgröße/1
  Kalman Filter1/1 -> Demux4/1
  Demux4/3 -> geschätzte Störgröße/1, Störgrößenaufschaltung1/1
  Umrechnung VZ Hub/1 -> Scope_n_Motor_Hub/1, DAC_Hub_Ansteuerung/1
  Störgrößenaufschaltung1/1 -> Sum6/1
  kalman_on/1(Out) -> Kalman Filter1/2
  "Initial State Geschwindigkeit, Störgröße"/1 -> Mux7/2
  Terminal/3(regler_an) -> Initial State/Trigger, kalman_on/Enable, Kalman Filter1/4, regler_on 4/1(regler_ on), regler_on 3/1(regler_ on), regler_on 1/1(regler_ on), regler_on 2/1(regler_ on), Kalman Filter/1(regler_an)
  Initial State/1(Out) -> Kalman Filter1/3
  Mux7/1 -> Initial State/1(In)
  yUout/1 -> ADC_yUout/1, Sum/2, Ausgangsgröße (Spannung)/1, Umrechnung VZ Hub1/1, Mux7/1, kalman_on/1(In)
  Umrechnung VZ Hub1/1 -> Sum5/1
  "Initial State Geschwindigkeit, Störgröße1"/1 -> Sum5/2
  Sum5/1 -> Kalman Filter/4(L)

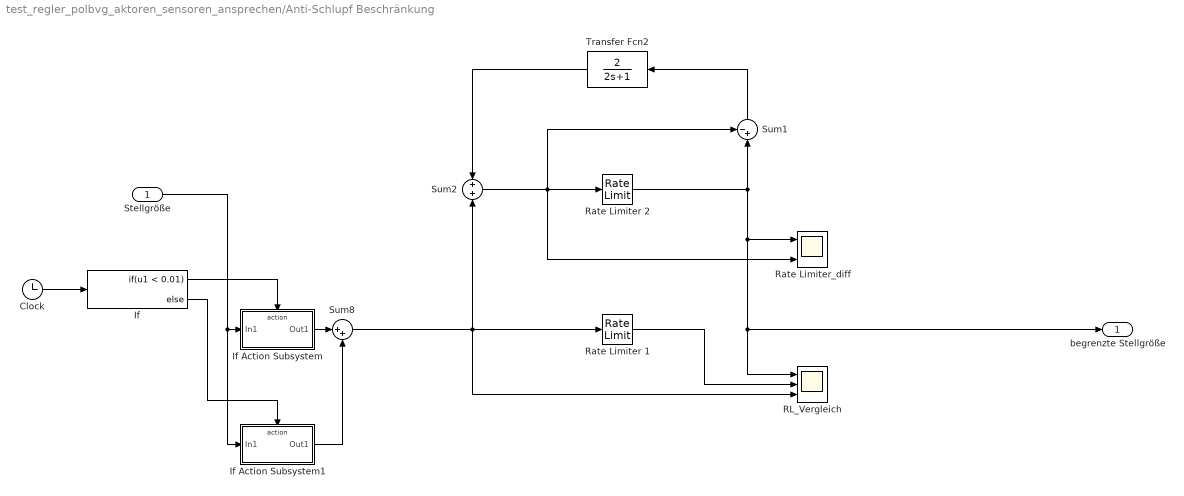
== system test_regler_polbvg_aktoren_sensoren_ansprechen/Anti-Schlupf Beschränkung ==
  Stellgröße : Inport
  Clock : Clock
  If : If  IfExpression=u1 < 0.01
  If Action Subsystem : Subsystem  TreatAsAtomicUnit=on
  If Action Subsystem1 : Subsystem  TreatAsAtomicUnit=on
  RL_Vergleich : Scope  NumInputPorts=3
  Rate Limiter 1 : RateLimiter  RisingSlewLimit=9.57  FallingSlewLimit=-9.57  SampleTimeMode=inherited
  Rate Limiter 2 : RateLimiter  RisingSlewLimit=9.57  FallingSlewLimit=-9.57  SampleTimeMode=inherited
  Rate Limiter_diff : Scope  NumInputPorts=2
  Sum1 : Sum  Inputs=-+|
  Sum2 : Sum  Inputs=+|+
  Sum8 : Sum  Inputs=|++
  Transfer Fcn2 : TransferFcn  Numerator=[2]  Denominator=[2 1]
  begrenzte Stellgröße : Outport
  wires:
  Stellgröße/1 -> If Action Subsystem1/1(In1), If Action Subsystem/1(In1)
  If Action Subsystem/1(Out1) -> Sum8/1
  If Action Subsystem1/1(Out1) -> Sum8/2
  Clock/1 -> If/1
  If/1 -> If Action Subsystem/Action
  If/2 -> If Action Subsystem1/Action
  Sum8/1 -> RL_Vergleich/3, Sum2/2, Rate Limiter 1/1
  Sum2/1 -> Rate Limiter_diff/2, Sum1/1, Rate Limiter 2/1
  Sum1/1 -> Transfer Fcn2/1
  Transfer Fcn2/1 -> Sum2/1
  Rate Limiter 2/1 -> begrenzte Stellgröße/1, RL_Vergleich/1, Rate Limiter_diff/1, Sum1/2
  Rate Limiter 1/1 -> RL_Vergleich/2

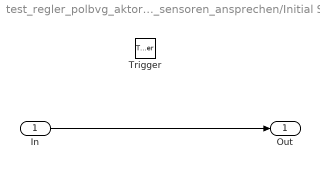
== system test_regler_polbvg_aktoren_sensoren_ansprechen/Initial State ==
  In : Inport
  Trigger : TriggerPort  VariantControl=Variant
  Out : Outport
  wires:
  In/1 -> Out/1

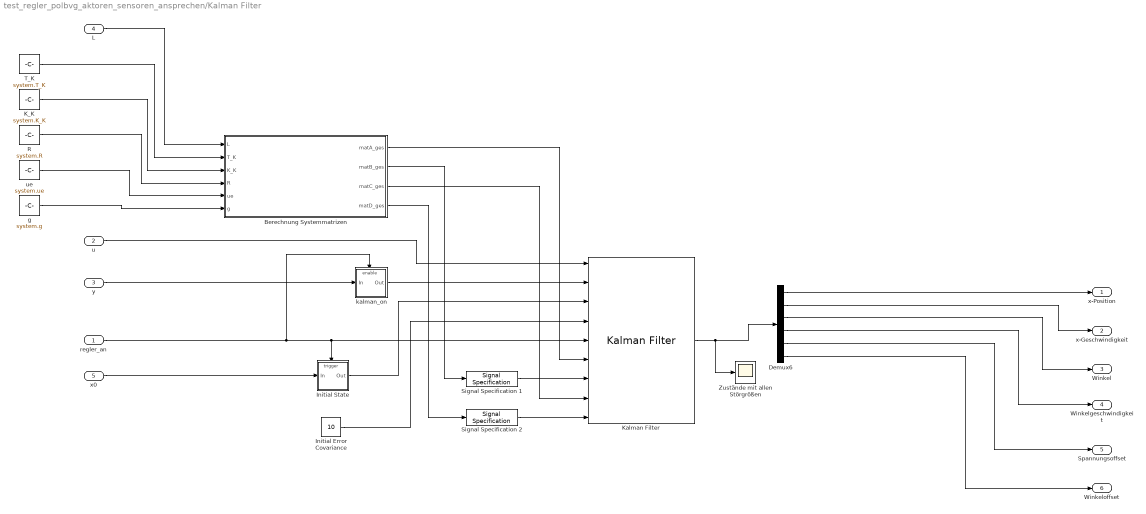
== system test_regler_polbvg_aktoren_sensoren_ansprechen/Kalman Filter ==
  regler_an : Inport
  u : Inport  Port=2
  y : Inport  Port=3
  L : Inport  Port=4
  x0 : Inport  Port=5
  Berechnung Systemmatrizen : MATLAB Function  TreatAsAtomicUnit=on
  Demux6 : Demux  Outputs=6
  Initial Error Covariance : Constant  Value=10
  Initial State : Subsystem  TreatAsAtomicUnit=on
  K_K : Constant  Value=system.K_K
  Kalman Filter : ctrlSharedLib/Kalman Filter  TimeDomain=Continuous-Time  UseCurrentEstimator=on  ModelSource=Input port  ModelSourceVariable=ss(0.95,1,1,0,1)  A=matA_g  B=matB_g  C=matC_g  D=0  NumberOfStates=6  NumberOfInputs=1  NumberOfOutputs=2  InitialEstimateSource=Input port  X0=0  P0=10  UseK=off  UseGH=on  NumberOfProcessNoiseInputs=1  G=matG_ges  TimeInvariantG=on  H=0  TimeInvariantH=on  Q=matQ_ges  TimeInvariantQ=on  R=matR_ges  TimeInvariantR=on  N=0  TimeInvariantN=on  AddInputPort=on  AddEnablePort=off  ExternalReset=rising  OutputEstimatedY=off  OutputP=off  Ts=-1
  R : Constant  Value=system.R
  Signal Specification 1 : SignalSpecification  Dimensions=[6 1]
  Signal Specification 2 : SignalSpecification  Dimensions=[2 1]
  T_K : Constant  Value=system.T_K
  Zustände mit allen Störgrößen : Scope
  g : Constant  Value=system.g
  kalman_on : Subsystem  TreatAsAtomicUnit=on
  ue : Constant  Value=system.ue
  x-Position : Outport
  x-Geschwindigkeit : Outport  Port=2
  Winkel : Outport  Port=3
  Winkelgeschwindigkeit : Outport  Port=4
  Spannungsoffset : Outport  Port=5
  Winkeloffset : Outport  Port=6
  wires:
  Demux6/5 -> Spannungsoffset/1
  u/1 -> Kalman Filter/1
  regler_an/1 -> kalman_on/Enable, Kalman Filter/5, Initial State/Trigger
  Demux6/1 -> x-Position/1
  Demux6/3 -> Winkel/1
  Demux6/4 -> Winkelgeschwindigkeit/1
  x0/1 -> Initial State/1(In)
  Demux6/6 -> Winkeloffset/1
  Demux6/2 -> x-Geschwindigkeit/1
  Berechnung Systemmatrizen/1(matA_ges) -> Kalman Filter/6
  Kalman Filter/1 -> Zustände mit allen Störgrößen/1, Demux6/1
  Berechnung Systemmatrizen/4(matD_ges) -> Signal Specification 2/1
  Berechnung Systemmatrizen/3(matC_ges) -> Kalman Filter/8
  kalman_on/1(Out) -> Kalman Filter/2
  Berechnung Systemmatrizen/2(matB_ges) -> Signal Specification 1/1
  Signal Specification 2/1 -> Kalman Filter/9
  L/1 -> Berechnung Systemmatrizen/1(L)
  Signal Specification 1/1 -> Kalman Filter/7
  y/1 -> kalman_on/1(In)
  Initial State/1(Out) -> Kalman Filter/3
  Initial Error Covariance/1 -> Kalman Filter/4
  g/1 -> Berechnung Systemmatrizen/6(g)
  ue/1 -> Berechnung Systemmatrizen/5(ue)
  R/1 -> Berechnung Systemmatrizen/4(R)
  K_K/1 -> Berechnung Systemmatrizen/3(K_K)
  T_K/1 -> Berechnung Systemmatrizen/2(T_K)

== system test_regler_polbvg_aktoren_sensoren_ansprechen/RTI Data ==
  RTI Data Store : Subsystem  Tag="struct('private',struct('version',struct('dsVer',uint32(2),'dsVerCreation',uint32(2),'RTI',struct('ver','7.7','type','RTI1202')),'access',struct('type','Model','isPerm',1,'created',['24-Nov-2020 10:16:32'],'modified',['02-Dec-2020 16:46:45'],'location','')),'public',struct('main',struct('data',[]),'sub',struct('name',{{'aktoren_sensoren_ansprechen'}},'data',{{struct('TH',struct('thTaskInfo',struct('taskType',{'TIMER','HWINT','TMRINT','SWINT','GLINT'},'tasksNumOf',{1,0,0,0,0},'srcIds',{{'TIMERA'},{},{},{},{}},'taskNames',{{['Timer Task 1']},{},{},{},{}})),'th_tc',struct('dataType','TASK','taskGroupId','','taskGroupList',{{}},'taskSchedulingPolicy','FCFS','taskType','TIMER','blkh',-1,'srcId','TIMERA','srcSgnName',['Timer A interrupt'],'srcCpuName','','taskName',['Timer Task 1  [0.001] s'],'taskNameDisplayExt','','smplTime',0.001,'smplTimeOffs',0,'hasFixedPriority',0,'priority',1,'hasFixedOvc',0,'ovcType',1,'ovcMax',1),'tc_th',struct('dataType','TASK','taskGroupId','','taskGroupList',{{}},'taskSchedulingPolicy','FCFS','taskType','TIMER','blkh',-1,'srcId','TIMERA','srcSgnName',['Timer A interrupt'],'srcCpuName','','taskName',['Timer Task 1  [0.001] s'],'taskNameDisplayExt','','smplTime',0.001,'smplTimeOffs',0,'hasFixedPriority',0,'priority',1,'hasFixedOvc',0,'ovcType',1,'ovcMax',1))}})))"  mask(RTI_DATA_STORE){}
      mask help:
      | RTI Data Store Block. This block is used by RTI to store internal model dependent data. Deleting this block will result in data loss.
      |
      | NEVER DELETE, COPY, OR MODIFY THIS BLOCK!
      mask Help:
      | RTI Data Store Block. This block is used by RTI to store internal model dependent data. Deleting this block will result in data loss.
      | 
      | NEVER DELETE, COPY, OR MODIFY THIS BLOCK!
      mask Display: text(0.5, 0.5, ' ', 'HorizontalAlignment', 'center');

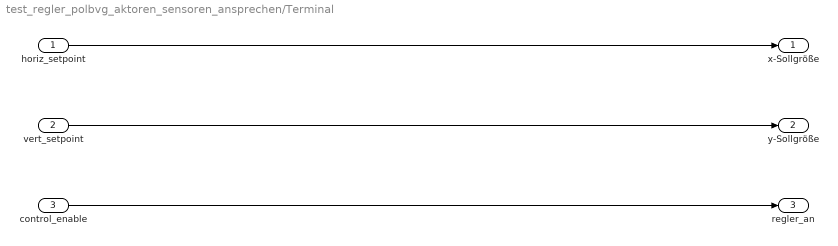
== system test_regler_polbvg_aktoren_sensoren_ansprechen/Terminal ==
  horiz_setpoint : Inport
  vert_setpoint : Inport  Port=2
  control_enable : Inport  Port=3
  x-Sollgröße : Outport
  y-Sollgröße : Outport  Port=2
  regler_an : Outport  Port=3
  wires:
  horiz_setpoint/1 -> x-Sollgröße/1
  vert_setpoint/1 -> y-Sollgröße/1
  control_enable/1 -> regler_an/1

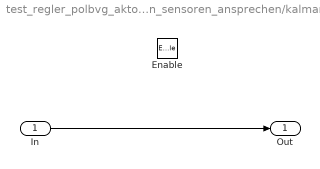
== system test_regler_polbvg_aktoren_sensoren_ansprechen/kalman_on ==
  In : Inport
  Enable : EnablePort
  Out : Outport
  wires:
  In/1 -> Out/1

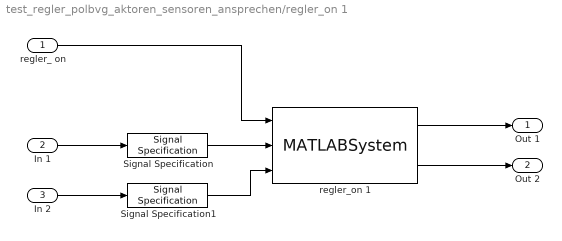
== system test_regler_polbvg_aktoren_sensoren_ansprechen/regler_on 1 ==
  regler_ on : Inport
  In 1 : Inport  Port=2
  In 2 : Inport  Port=3
  Signal Specification : SignalSpecification  Dimensions=1
  Signal Specification1 : SignalSpecification  Dimensions=1
  regler_on 1 : MATLABSystem  System=regler_switch_2  SimulateUsing=Code generation
      mask Type: regler_switch_2
      mask Display:
      | disp('regler_switch_2');
      | port_label('input',1,'regler_on');
      | port_label('input',2,'input1');
      | port_label('input',3,'input2');
      | port_label('output',1,'y1');
      | port_label('output',2,'y2');
  Out 1 : Outport
  Out 2 : Outport  Port=2
  wires:
  regler_on 1/1 -> Out 1/1
  regler_on 1/2 -> Out 2/1
  In 2/1 -> Signal Specification1/1
  In 1/1 -> Signal Specification/1
  Signal Specification/1 -> regler_on 1/2
  Signal Specification1/1 -> regler_on 1/3
  regler_ on/1 -> regler_on 1/1

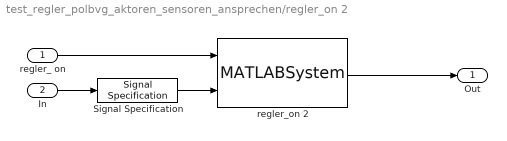
== system test_regler_polbvg_aktoren_sensoren_ansprechen/regler_on 2 ==
  regler_ on : Inport
  In : Inport  Port=2
  Signal Specification : SignalSpecification  Dimensions=1
  regler_on 2 : MATLABSystem  System=regler_switch_1  SimulateUsing=Code generation
      mask Type: regler_switch_1
      mask Display:
      | disp('regler_switch_1');
      | port_label('input',1,'regler_on');
      | port_label('input',2,'input');
      | port_label('output',1,'y');
  Out : Outport
  wires:
  regler_ on/1 -> regler_on 2/1
  regler_on 2/1 -> Out/1
  Signal Specification/1 -> regler_on 2/2
  In/1 -> Signal Specification/1

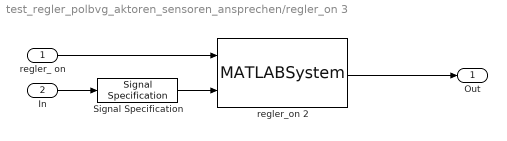
== system test_regler_polbvg_aktoren_sensoren_ansprechen/regler_on 3 ==
  regler_ on : Inport
  In : Inport  Port=2
  Signal Specification : SignalSpecification  Dimensions=1
  regler_on 2 : MATLABSystem  System=regler_switch_1  SimulateUsing=Code generation
      mask Type: regler_switch_1
      mask Display:
      | disp('regler_switch_1');
      | port_label('input',1,'regler_on');
      | port_label('input',2,'input');
      | port_label('output',1,'y');
  Out : Outport
  wires:
  regler_ on/1 -> regler_on 2/1
  regler_on 2/1 -> Out/1
  Signal Specification/1 -> regler_on 2/2
  In/1 -> Signal Specification/1

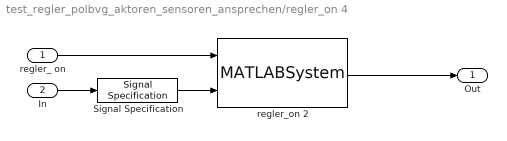
== system test_regler_polbvg_aktoren_sensoren_ansprechen/regler_on 4 ==
  regler_ on : Inport
  In : Inport  Port=2
  Signal Specification : SignalSpecification  Dimensions=1
  regler_on 2 : MATLABSystem  System=regler_switch_1  SimulateUsing=Code generation
      mask Type: regler_switch_1
      mask Display:
      | disp('regler_switch_1');
      | port_label('input',1,'regler_on');
      | port_label('input',2,'input');
      | port_label('output',1,'y');
  Out : Outport
  wires:
  regler_ on/1 -> regler_on 2/1
  regler_on 2/1 -> Out/1
  Signal Specification/1 -> regler_on 2/2
  In/1 -> Signal Specification/1

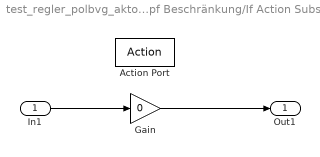
== system test_regler_polbvg_aktoren_sensoren_ansprechen/Anti-Schlupf Beschränkung/If Action Subsystem ==
  In1 : Inport
  Action Port : ActionPort
  Gain : Gain  Gain=0
  Out1 : Outport
  wires:
  In1/1 -> Gain/1
  Gain/1 -> Out1/1

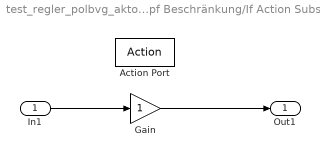
== system test_regler_polbvg_aktoren_sensoren_ansprechen/Anti-Schlupf Beschränkung/If Action Subsystem1 ==
  In1 : Inport
  Action Port : ActionPort
  Gain : Gain
  Out1 : Outport
  wires:
  In1/1 -> Gain/1
  Gain/1 -> Out1/1

== system test_regler_polbvg_aktoren_sensoren_ansprechen/Kalman Filter/Initial State ==
  In : Inport
  Trigger : TriggerPort  VariantControl=Variant
  Out : Outport
  wires:
  In/1 -> Out/1

== system test_regler_polbvg_aktoren_sensoren_ansprechen/Kalman Filter/kalman_on ==
  In : Inport
  Enable : EnablePort
  Out : Outport
  wires:
  In/1 -> Out/1

== system test_regler_polbvg_aktoren_sensoren_ansprechen/RTI Data/RTI Data Store ==
  RTI Data Store : Subsystem  mask(RTI_DATA_STORE){}
      mask help:
      | RTI Data Store Block. This block is used by RTI to store internal model dependent data. Deleting this block will result in data loss.
      |
      | NEVER DELETE, COPY, OR MODIFY THIS BLOCK!
      mask Help:
      | RTI Data Store Block. This block is used by RTI to store internal model dependent data. Deleting this block will result in data loss.
      | 
      | NEVER DELETE, COPY, OR MODIFY THIS BLOCK!
      mask Display: text(0.5, 0.5, ' ', 'HorizontalAlignment', 'center');
